simulink model "cap"  (R2024a)
settings: Solver=FixedStepDiscrete  StartTime=0.0  StopTime=5  FixedStep=10e-6  RelTol=1e-3
libraries: spsSeriesRLCBranchLib x4, spsCurrentMeasurementLib x2, simulink x2, spsVoltageMeasurementLib x2, spsDiodeLib x1, spsIGBTDiodeLib x1, spsPVArrayLib x1, spsPWMGeneratorDCDCLib x1, spspowerguiLib x1
settings Model: Creator=HP  LastModifiedBy=huangz

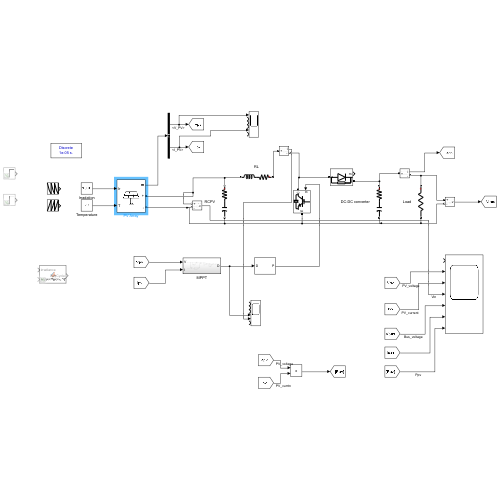
[thumbnail: Simulink's stored preview of the top-level diagram]
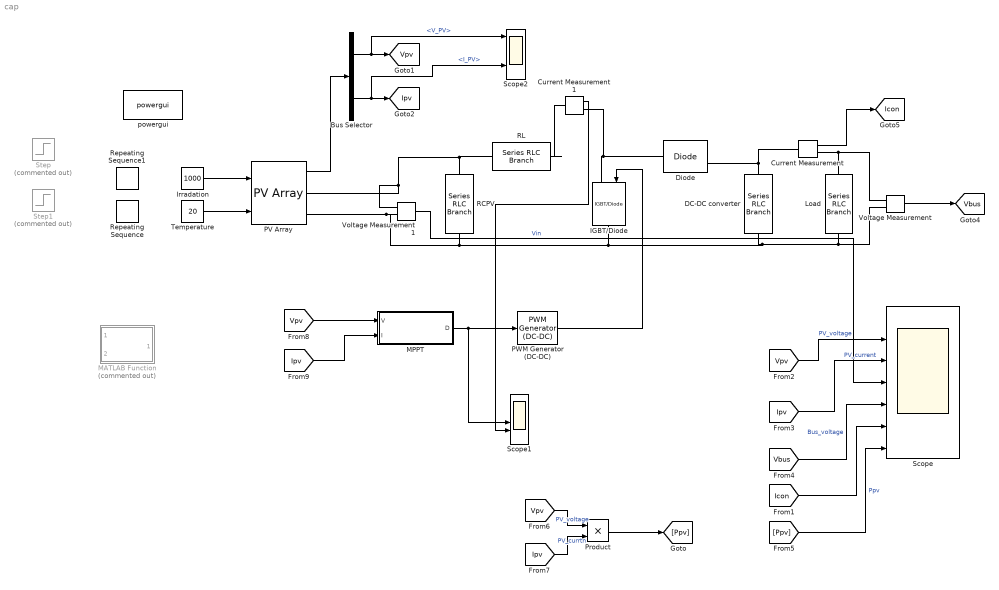
== system cap ==
  Bus Selector : BusSelector  OutputSignals=V_PV,I_PV
  Current Measurement : spsCurrentMeasurementLib/Current Measurement  PhasorSimulation=off  OutputType=Complex  PSBequivalent=0
  Current Measurement1 : spsCurrentMeasurementLib/Current Measurement  PhasorSimulation=off  OutputType=Complex  PSBequivalent=0
  DC-DC converter : spsSeriesRLCBranchLib/Series RLC Branch  LConnTagsString=__new0  RConnTagsString=__new0  BranchType=RC  Resistance=1e-10  Inductance=1e-3  SetiL0=off  InitialCurrent=0  Capacitance=3300e-6  Setx0=off  InitialVoltage=0  Measurements=None
  Diode : spsDiodeLib/Diode  Ron=1e-10  Lon=0  Vf=1e-10  IC=0  UseSnubber=0  Rs=500  Cs=250e-9  Measurements=on
  IGBT/Diode : spsIGBTDiodeLib/IGBT//Diode  Ron=1e-10  Rs=1e5  Cs=inf  Measurements=off
  Irradation : Constant  Value=1000
  Load : spsSeriesRLCBranchLib/Series RLC Branch  LConnTagsString=__new0  RConnTagsString=__new0  BranchType=R  Resistance=8.5  Inductance=1e-3  SetiL0=off  InitialCurrent=0  Capacitance=3300e-6  Setx0=off  InitialVoltage=0  Measurements=None
  MATLAB Function : MATLAB Function  Commented=on  TreatAsAtomicUnit=on
  MPPT : Subsystem
  PV Array : spsPVArrayLib/PV Array  Npar=2  Nser=1  PlotType=array @ 25 deg.C & specified irradiances  S_vec="[ 1000  800  600 400 200 ]"  Temp_C_vec=20  ModuleName=Advance Power API-M300  PlotWhenSelected=off  Pm=300.0024  Ncell=72  Voc=44.71  Isc=8.58  Vm=36.72  Im=8.17  beta_Voc_pc=-0.3244  alpha_Isc_pc=0.053322  beta_Voc=-0.14504  alpha_Isc=0.004575  IL=8.6047  I0=7.8609e-11  nI=0.95103  Rsh=1116.1662  Rs=0.32911  RobustModel=off  RobustCellTemperature=313.3991  BAL=on  Tc=1e-6  Tfilter=5e-5
  PWM Generator (DC-DC) : spsPWMGeneratorDCDCLib/PWM Generator (DC-DC)  Fsw=25000  Ts=0
  Product : Product
  RCPV : spsSeriesRLCBranchLib/Series RLC Branch  LConnTagsString=__new0  RConnTagsString=__new0  BranchType=RC  Resistance=1e-10  Inductance=1e-3  SetiL0=off  InitialCurrent=0  Capacitance=350e-6  Setx0=off  InitialVoltage=0  Measurements=None
  RL : spsSeriesRLCBranchLib/Series RLC Branch  LConnTagsString=__new0  RConnTagsString=__new0  BranchType=RL  Resistance=1e-10  Inductance=120e-3  SetiL0=off  InitialCurrent=0  Capacitance=100e-6  Setx0=off  InitialVoltage=0  Measurements=None
  Repeating Sequence : simulink/Sources/Repeating Sequence  rep_seq_t=[0 2.5 5]  rep_seq_y=[20 30 40]
  Repeating Sequence1 : simulink/Sources/Repeating Sequence  rep_seq_t=[0 1 2]  rep_seq_y=[1000 600 400]
  Scope : Scope  NumInputPorts=7
  Scope1 : Scope  NumInputPorts=6
  Scope2 : Scope  NumInputPorts=6
  Step : Step  Commented=on  Time=2.5  Before=800  After=1000  SampleTime=0
  Step1 : Step  Commented=on  Time=2.5  Before=20  After=40  SampleTime=0
  Temperature : Constant  Value=20
  Voltage Measurement : spsVoltageMeasurementLib/Voltage Measurement  PhasorSimulation=off  OutputType=Complex  PSBequivalent=0
  Voltage Measurement1 : spsVoltageMeasurementLib/Voltage Measurement  PhasorSimulation=off  OutputType=Complex  PSBequivalent=0
  powergui : spspowerguiLib/powergui  Priority=1  SimulationMode=Discrete  SampleTime=10e-6  frequency=60  Iterations=50  frequencyindice=0  Pbase=100e6  ErrMax=1e-4  UnitsV=kV  UnitsW=MW  buscounter=0  FunctionMessages=off  echomessages=off  EnableUseOfTLC=off  CurrentSourceSwitches=off  DisableSnubberDevices=off  DisableRonSwitches=off  DisableVfSwitches=off  DisplayEquations=off  AutomaticDiscreteSolvers=off  SolverType=Tustin/Backward Euler (TBE)  Interpol=off  ExternalGateDelay=off  methode=off  Ts=100  x0status=blocks  SPID=on  SwTol=0  HookPort=off  NonlinearTolerance=1e-4  nMaxIteration=100  ContinueOnMaxIteration=off  RestoreLinks=warning  ResistiveCurrentMeasurement=off  Frange=[0:2:500]  Ylog=off  Xlog=on  ShowGrid=off  save=off  variable=ZData  structure=0  ZoomFFT=off  StartTime=0.0  cycles=1  DisplayStyle=1  fundamental=60  FreqAxis=off  MaxFrequency=1000  frequencyindicesteady=1  RmsSteady=1  display=off
  tag scope: Icon=global, Ipv=global, Vbus=global, Vpv=global
  wires:
  PV Array/1 -> Bus Selector/1
  Bus Selector/1 -> Scope2/1, [Vpv]  "<V_PV>"
  Bus Selector/2 -> Scope2/5, [Ipv]  "<I_PV>"
  Current Measurement/1 -> [Icon]
  [Vpv] -> Scope/2  "PV_voltage"
  [Ipv] -> Scope/3  "PV_current"
  Voltage Measurement/1 -> [Vbus]
  [Vbus] -> Scope/5  "Bus_voltage"
  [Icon] -> Scope/6
  [Ppv] -> Scope/7  "Ppv"
  Product/1 -> [Ppv]
  [Vpv] -> Product/1  "PV_voltage"
  [Ipv] -> Product/2  "PV_currtn"
  [Vpv] -> MPPT/1(V)
  [Ipv] -> MPPT/2(I)
  PWM Generator (DC-DC)/1 -> IGBT/Diode/1
  Voltage Measurement1/1 -> Scope/4  "Vin"
  Current Measurement1/1 -> Scope1/5
  MPPT/1(D) -> Scope1/4, PWM Generator (DC-DC)/1
  Temperature/1 -> PV Array/2
  Irradation/1 -> PV Array/1
  connections:
  PV Array/RConn1 -- RCPV/LConn1 -- RL/RConn1 -- Voltage Measurement1/LConn1
  PV Array/RConn2 -- Voltage Measurement/LConn2 -- Load/RConn1 -- DC-DC converter/RConn1 -- IGBT/Diode/RConn1 -- RCPV/RConn1 -- Voltage Measurement1/LConn2
  Diode/LConn1 -- Current Measurement1/RConn1 -- IGBT/Diode/LConn1
  Current Measurement/RConn1 -- Load/LConn1 -- Voltage Measurement/LConn1
  Diode/RConn1 -- Current Measurement/LConn1 -- DC-DC converter/LConn1
  RL/LConn1 -- Current Measurement1/LConn1

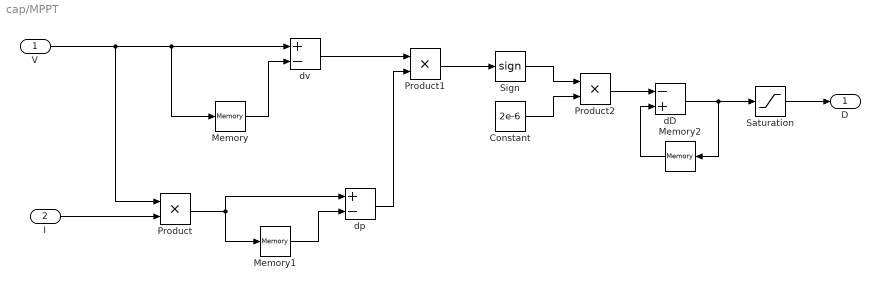
== system cap/MPPT ==
  V : Inport
  I : Inport  Port=2
  Constant : Constant  Value=2e-6
  Memory : Memory
  Memory1 : Memory
  Memory2 : Memory  InitialCondition=0.52
  Product : Product
  Product1 : Product
  Product2 : Product
  Saturation : Saturate  UpperLimit=0.95  LowerLimit=0.1
  Sign : Signum
  dD : Sum  Inputs=-+
  dp : Sum  Inputs=+-
  dv : Sum  Inputs=+-
  D : Outport
  wires:
  I/1 -> Product/2
  V/1 -> Product/1, Memory/1, dv/1
  Memory/1 -> dv/2
  dv/1 -> Product1/1
  Product/1 -> dp/1, Memory1/1
  Memory1/1 -> dp/2
  dp/1 -> Product1/2
  Product1/1 -> Sign/1
  Sign/1 -> Product2/1
  Constant/1 -> Product2/2
  Product2/1 -> dD/1
  Memory2/1 -> dD/2
  dD/1 -> Saturation/1, Memory2/1
  Saturation/1 -> D/1

== matlab function cap/MATLAB Function ==
  data: irradiance input; dutyCycle output; temperature input
function dutyCycle = decisionTreeMPPT(irradiance, temperature)
